simulink model "Variable_PID_ANN_gain_selector"  (R2020a)
settings: Solver=VariableStepAuto  StartTime=0.0  StopTime=0.08  RelTol=1e-3
undefined symbols (not defined in the file or in its folder): Ion, Lithium
libraries: neural x30, powerlib x15, simulink x3, powerlib_meascontrol x3, eeStairGenerator x3, electricdrivelib x1, re_lib x1
(part 2 of 2)

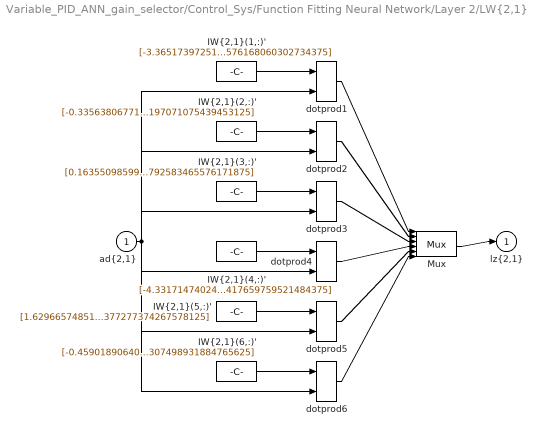
== system Variable_PID_ANN_gain_selector/Control_Sys/Function Fitting Neural Network/Layer 2/LW{2,1} ==
  "ad{2,1}" : Inport  PortDimensions=20
      mask Display: e = 0.06;c1 = [120 230 180]/255;c2 = ([120 230 180]+0)/(256+128);c3 = ([120 230 180]+128)/(256+128);patch([0 1 1 0],[0 0 1 1],c1);patch([0 1 1 1-e 1-e 0+e],[0 0 1 1-e 0+e 0+e],c2);patch([0 0 1 1-e 0+e 0+e],[0 1 1 1-e 1-e 0+e],c3);plot([0 1 1 0 0],[0 0 1 1 0]);
  "IW{2,1}(1,:)'" : Constant  Value=[-3.36517397251916872136234815116040408611297607421875;0.65428202037868121720975977950729429721832275390625;6.6071855148608751306937847402878105640411376953125;-0.0978931999035662359087694994741468690335750579833984375;-1.307015964313751776870731191593222320079803466796875;1.6896653097461811210422411022591404616832733154296875;0.6320520445307618029318064145627431571483612060546875;1.6045864139040253437684668824658729135990142822265625;2.36865100396856664843880935222841799259185791015625;-0.11212521566580525844702975746258744038641452789306640625;3.1372657907513659125697813578881323337554931640625;0.0539010546169985949038760963958338834345340728759765625;-1.2050343651996213711896643872023560106754302978515625;-2.492746828485352228454985379357822239398956298828125;3.793253251905604361837731630657799541950225830078125;-0.9641072843967812833199104716186411678791046142578125;-0.89666534518325846647712751291692256927490234375;-0.640674643417033617964762015617452561855316162109375;3.436337450050871655804485271801240742206573486328125;2.8007173489256640408484599902294576168060302734375]
      mask Display: e = 0.06;c1 = [120 150 230]/255;c2 = ([120 150 230]+0)/383;c3 = ([120 150 230]+128)/383;patch([0 1 1 0],[0 0 1 1],c1);patch([0 1 1 1-e 1-e 0+e],[0 0 1 1-e 0+e 0+e],c2);patch([0 0 1 1-e 0+e 0+e],[0 1 1 1-e 1-e 0+e],c3);plot([0 1 1 0 0],[0 0 1 1 0]);disp('weights');
  "IW{2,1}(2,:)'" : Constant  Value=[-0.3356380677146404423183412291109561920166015625;0.29563870064403641180206250282935798168182373046875;0.1930359420841606665764089711956330575048923492431640625;0.18882099354445325278817335856729187071323394775390625;0.3386678091089887487896703532896935939788818359375;0.0540247173621271059573700767941772937774658203125;-0.07039064675486654543146158857780392281711101531982421875;1.023370826575114467260618766886182129383087158203125;1.379272547700930662273322013788856565952301025390625;-0.345349393753670186324455926296650432050228118896484375;-0.271941842749966078418566439722781069576740264892578125;0.0479471242757519566790591625249362550675868988037109375;-0.822794290911861292414641866344027221202850341796875;-0.232392377536564331830248875121469609439373016357421875;1.1190743246650403097675052777049131691455841064453125;-0.97771308145563728952964765994693152606487274169921875;-0.35923001890646244493865424374234862625598907470703125;-0.79212214166073879884066855083801783621311187744140625;4.37417571572724028783341054804623126983642578125;3.077074203356023218702830490656197071075439453125]
      mask Display: e = 0.06;c1 = [120 150 230]/255;c2 = ([120 150 230]+0)/383;c3 = ([120 150 230]+128)/383;patch([0 1 1 0],[0 0 1 1],c1);patch([0 1 1 1-e 1-e 0+e],[0 0 1 1-e 0+e 0+e],c2);patch([0 0 1 1-e 0+e 0+e],[0 1 1 1-e 1-e 0+e],c3);plot([0 1 1 0 0],[0 0 1 1 0]);disp('weights');
  "IW{2,1}(3,:)'" : Constant  Value=[0.1635509859917323727263038790624705143272876739501953125;-0.2103157068725303446843355459350277669727802276611328125;-1.0767935612704497838620909533347003161907196044921875;-0.400893366144898621872272315158625133335590362548828125;-1.279980228460594116057791325147263705730438232421875;0.70370204684158166319463134641409851610660552978515625;0.259085526014026956698188541849958710372447967529296875;-0.52103435900761352339571885750046931207180023193359375;-1.316399237038669678412361463415436446666717529296875;0.4881341980643576494713897773181088268756866455078125;2.029702220857416694599351103533990681171417236328125;-0.0646919259421786796426800947301671840250492095947265625;0.8495872954939571730648140146513469517230987548828125;1.229222791803018299816585567896254360675811767578125;-1.970482821074982293652055886923335492610931396484375;0.8023815728278227421554902321076951920986175537109375;0.450609678929167534189303978564566932618618011474609375;0.5647421235761413971232514086295850574970245361328125;-3.452846633904059547859333179076202213764190673828125;-3.142811136660227600003736370126716792583465576171875]
      mask Display: e = 0.06;c1 = [120 150 230]/255;c2 = ([120 150 230]+0)/383;c3 = ([120 150 230]+128)/383;patch([0 1 1 0],[0 0 1 1],c1);patch([0 1 1 1-e 1-e 0+e],[0 0 1 1-e 0+e 0+e],c2);patch([0 0 1 1-e 0+e 0+e],[0 1 1 1-e 1-e 0+e],c3);plot([0 1 1 0 0],[0 0 1 1 0]);disp('weights');
  "IW{2,1}(4,:)'" : Constant  Value=[-4.331714740245754313718862249515950679779052734375;2.991313526877215966948142522596754133701324462890625;10.2351488754831994043570375652052462100982666015625;4.38260152656374657453852705657482147216796875;4.35042434990471260647382223396562039852142333984375;-5.03495306506535822421710690832696855068206787109375;-2.21358884779430820088919062982313334941864013671875;1.594588767979347121439559487043879926204681396484375;1.4215108509988729768025450539425946772098541259765625;-0.708473493324877079402313029277138411998748779296875;-9.836020919024118569495840347371995449066162109375;-0.068734176246332212567580199902295134961605072021484375;1.1652670520466148484928226025658659636974334716796875;-0.10152427409112081690967244185230811126530170440673828125;0.99600776883887987001031660838634707033634185791015625;2.816934877029288575300824959413148462772369384765625;-0.66376888781892151580876770822214893996715545654296875;2.625366424137961285367737218621186912059783935546875;7.777154900430549133716340293176472187042236328125;8.1884154360741003841894780634902417659759521484375]
      mask Display: e = 0.06;c1 = [120 150 230]/255;c2 = ([120 150 230]+0)/383;c3 = ([120 150 230]+128)/383;patch([0 1 1 0],[0 0 1 1],c1);patch([0 1 1 1-e 1-e 0+e],[0 0 1 1-e 0+e 0+e],c2);patch([0 0 1 1-e 0+e 0+e],[0 1 1 1-e 1-e 0+e],c3);plot([0 1 1 0 0],[0 0 1 1 0]);disp('weights');
  "IW{2,1}(5,:)'" : Constant  Value=[1.6296657485147514332624041344388388097286224365234375;0.56110338799388481678676043884479440748691558837890625;-0.6522257847681334208544967623311094939708709716796875;-0.52920871021113580212613669573329389095306396484375;-0.169125650872955279879761292249895632266998291015625;1.2244930515755341193795402432442642748355865478515625;-0.07961088221061439484937949373488663695752620697021484375;0.11833790590850490342944567601080052554607391357421875;-0.00596192432720968161496966075674208696000277996063232421875;-0.2490420302723544143663758632101234979927539825439453125;1.404654396087268164450279073207639157772064208984375;0.0930122295749757632687959585382486693561077117919921875;0.1830527632635965407104094992973841726779937744140625;0.09644571343541928631903914492795593105256557464599609375;-0.0902739886805592195440084424262749962508678436279296875;0.417654600163804901047370776723255403339862823486328125;-0.03987113761589532179296924141453928314149379730224609375;0.37931939703750305881158055854029953479766845703125;0.5299801143903357658615504988119937479496002197265625;0.85284209571151514683862160381977446377277374267578125]
      mask Display: e = 0.06;c1 = [120 150 230]/255;c2 = ([120 150 230]+0)/383;c3 = ([120 150 230]+128)/383;patch([0 1 1 0],[0 0 1 1],c1);patch([0 1 1 1-e 1-e 0+e],[0 0 1 1-e 0+e 0+e],c2);patch([0 0 1 1-e 0+e 0+e],[0 1 1 1-e 1-e 0+e],c3);plot([0 1 1 0 0],[0 0 1 1 0]);disp('weights');
  "IW{2,1}(6,:)'" : Constant  Value=[-0.459018906400530612987864742535748519003391265869140625;1.6163977786727452556903017466538585722446441650390625;3.433229120911255538572959267185069620609283447265625;0.735020594500215285194144598790444433689117431640625;1.0287916357919240084584089345298707485198974609375;-0.1817950475947720800906637350635719485580921173095703125;-0.52682269774995071909273747223778627812862396240234375;0.92981230838954853634703567877295427024364471435546875;0.7613790755285931854956515962840057909488677978515625;-0.459348638545453435977350409302744083106517791748046875;-1.2946504218855989787329008322558365762233734130859375;0.08249383763885632936396774539389298297464847564697265625;0.144804628516190081466419314892846159636974334716796875;-0.31958024062859313740858624441898427903652191162109375;0.7832308147794446728795492163044400513172149658203125;0.478123821064538656600007016095332801342010498046875;-0.29838661729146076506680174134089611470699310302734375;0.479401783375590750946315665714791975915431976318359375;2.834624493187036353702978885849006474018096923828125;2.57008407532405414031018153764307498931884765625]
      mask Display: e = 0.06;c1 = [120 150 230]/255;c2 = ([120 150 230]+0)/383;c3 = ([120 150 230]+128)/383;patch([0 1 1 0],[0 0 1 1],c1);patch([0 1 1 1-e 1-e 0+e],[0 0 1 1-e 0+e 0+e],c2);patch([0 0 1 1-e 0+e 0+e],[0 1 1 1-e 1-e 0+e],c3);plot([0 1 1 0 0],[0 0 1 1 0]);disp('weights');
  Mux : Mux  Inputs=6
      mask Display: e = 0.06;c1 = [120 150 230]/255;c2 = ([120 150 230]+0)/383;c3 = ([120 150 230]+128)/383;patch([0 1 1 0],[0 0 1 1],c1);patch([0 1 1 1-e 1-e 0+e],[0 0 1 1-e 0+e 0+e],c2);patch([0 0 1 1-e 0+e 0+e],[0 1 1 1-e 1-e 0+e],c3);plot([0 1 1 0 0],[0 0 1 1 0]);disp('Mux');
  dotprod{1..6} (6 alike) : neural/Weight Functions/dotprod
  "lz{2,1}" : Outport
      mask Display: e = 0.06;c1 = [120 230 180]/255;c2 = ([120 230 180]+0)/(256+128);c3 = ([120 230 180]+128)/(256+128);patch([0 1 1 0],[0 0 1 1],c1);patch([0 1 1 1-e 1-e 0+e],[0 0 1 1-e 0+e 0+e],c2);patch([0 0 1 1-e 0+e 0+e],[0 1 1 1-e 1-e 0+e],c3);plot([0 1 1 0 0],[0 0 1 1 0]);
  wires:
  "IW{2,1}(1,:)'"/1 -> dotprod1/1
  "ad{2,1}"/1 -> dotprod1/2, dotprod2/2, dotprod3/2, dotprod4/2, dotprod5/2, dotprod6/2
  dotprod1/1 -> Mux/1
  "IW{2,1}(2,:)'"/1 -> dotprod2/1
  dotprod2/1 -> Mux/2
  "IW{2,1}(3,:)'"/1 -> dotprod3/1
  dotprod3/1 -> Mux/3
  "IW{2,1}(4,:)'"/1 -> dotprod4/1
  dotprod4/1 -> Mux/4
  "IW{2,1}(5,:)'"/1 -> dotprod5/1
  dotprod5/1 -> Mux/5
  "IW{2,1}(6,:)'"/1 -> dotprod6/1
  dotprod6/1 -> Mux/6
  Mux/1 -> "lz{2,1}"/1

== matlab function Variable_PID_ANN_gain_selector/Control_Sys/MATLAB Function ==
  data: I_pvf input; I_norm output; V_rf input; I_rf input; R_norm output
function [I_norm,R_norm] = fcn(I_pvf,V_rf,I_rf)
    if I_pvf==0
        R_norm=20;
    else
        R_norm=V_rf/I_rf;
    end
    %Adjust limits of R
    if R_norm>20
        R_norm=20;
    end
    if R_norm<1
        R_norm=1;
    end
    I_norm=(I_pvf/66.22)-0.5;
    R_norm=(R_norm/20)-0.5;
